simulink model "LQR_probleme_de_urmarire_cu_integrator"  (R2023b)
settings: Solver=VariableStepAuto  StartTime=0.0  StopTime=100  RelTol=1e-3
values from neighbouring files (symbols this model uses):
  A = [0 lambda 0 0 ... (first row only)    [rotary_inverted_pendulum.m]    (also in sis_liniar.m)
  B = [0; B21; 0; B41]./lambda    [rotary_inverted_pendulum.m]    (also in sis_liniar.m)
  C = [0 0 1 0]    [rotary_inverted_pendulum.m]
  Kx = K(1:4)    [rotary_inverted_pendulum.m]
  Kz = K(5)    [rotary_inverted_pendulum.m]
settings Model: Creator=ovidiuceoca  LastModifiedBy=ovidiuceoca

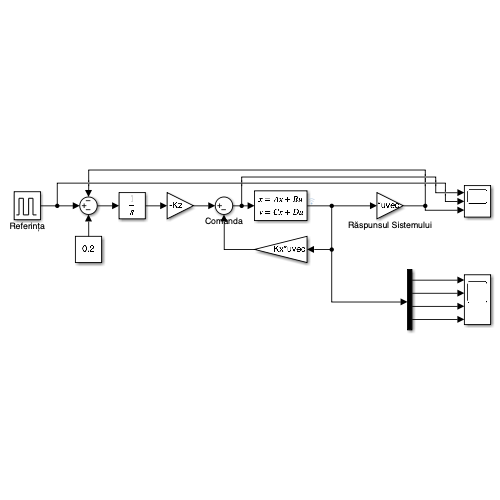
[thumbnail: Simulink's stored preview of the top-level diagram]
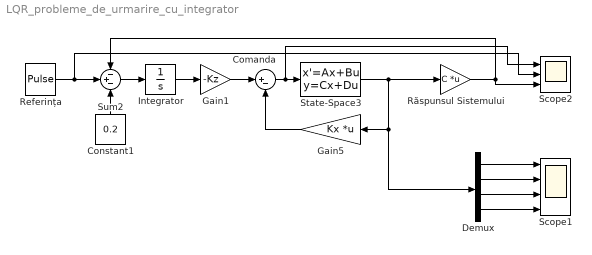
== system LQR_probleme_de_urmarire_cu_integrator ==
  Comanda : Sum  Inputs=|+-
  Constant1 : Constant  Value=0.2
  Demux : Demux
  Gain1 : Gain  Gain=-Kz
  Gain5 : Gain  Gain=Kx  Multiplication=Matrix(K*u) (u vector)
  Integrator : Integrator
  Referința : DiscretePulseGenerator  PulseType=Time based  Amplitude=0.4  Period=30  PulseWidth=50  PhaseDelay=15
  Răspunsul Sistemului : Gain  Gain=C  Multiplication=Matrix(K*u) (u vector)
  Scope1 : Scope  NumInputPorts=4
  Scope2 : Scope  NumInputPorts=3
  State-Space3 : StateSpace  A=A  B=B  C=eye(4)  D=[0;0;0;0]  InitialCondition=[1;1;1;1]
  Sum2 : Sum  Inputs=-+-
  wires:
  Comanda/1 -> Scope2/1, State-Space3/1
  State-Space3/1 -> Gain5/1, Demux/1, Răspunsul Sistemului/1
  Gain5/1 -> Comanda/2
  Referința/1 -> Scope2/2, Sum2/2
  Constant1/1 -> Sum2/3
  Integrator/1 -> Gain1/1
  Sum2/1 -> Integrator/1
  Gain1/1 -> Comanda/1
  Răspunsul Sistemului/1 -> Sum2/1, Scope2/3
  Demux/1 -> Scope1/1
  Demux/2 -> Scope1/2
  Demux/3 -> Scope1/3
  Demux/4 -> Scope1/4
